simulink model "modello_completo_simulink2019b"  (R2019b)
settings: Solver=VariableStepAuto  StartTime=0.0  StopTime=30  RelTol=1e-3
undefined symbols (not defined in the file): a, a1, a2, AHRS_bias, AHRS_sample_time, AHRS_var, alpha1, alpha2, c, current, D, dead_zone_limit, DiscIntNeverNeededParam, DVL_sample_t, DVL_var1, DVL_var2, DVL_var3, gps_sample_t, H, IMU_sample_time, initial, INSP, Ki_bodypos1, Ki_bodypos2, Ki_bodypos3, Ki_bodypos4, Ki_bodypos5, Ki_depth1, Ki_depth2, Ki_depth3, Ki_depth4, Ki_depth5, Ki_latvel1, Ki_latvel2, Ki_latvel3, Ki_latvel4, Ki_latvel5, Ki_P1, Ki_P2, Ki_P3, Ki_P4, Ki_P5, Ki_R1, Ki_R2, Ki_R3, Ki_R4, Ki_R5, Ki_rel_or1, Ki_rel_or2, Ki_rel_or3, Ki_rel_or4, Ki_rel_or5, Ki_reldist1, Ki_reldist2, Ki_reldist3, Ki_reldist4, Ki_reldist5, Ki_surge1, Ki_surge2, Ki_surge3 ... (+66)
libraries: simulink x3
(part 4 of 5)

== system modello_completo_simulink2019b/Controller/POSIZIONAMENTO/PID_PITCH ==
  pitch_err : Inport
  EN6 : Inport  Port=2
  Constant : Constant  Value=0
  Discrete-Time Integrator : DiscreteIntegrator  ExternalReset=falling  SampleTime=0.1  ICPrevOutput=DiscIntNeverNeededParam  ICPrevScaledInput=DiscIntNeverNeededParam
  Display : Display
  Display1 : Display
  Gain : Gain  Gain=Kp_P1
  Gain2 : Gain  Gain=Ki_P1
  Sum : Sum  Inputs=++|
  Switch : Switch  Criteria=u2 > Threshold  Threshold=0.5
  tau_pitch : Outport
  wires:
  Switch/1 -> Gain/1, Gain2/1
  Constant/1 -> Switch/3
  EN6/1 -> Display/1, Switch/2, [EN6]
  pitch_err/1 -> Switch/1
  Gain/1 -> Sum/1
  Discrete-Time Integrator/1 -> Sum/2
  Sum/1 -> Display1/1, tau_pitch/1
  Gain2/1 -> Discrete-Time Integrator/1
  [EN6] -> Discrete-Time Integrator/2

== system modello_completo_simulink2019b/Controller/POSIZIONAMENTO/PID_ROLL  ==
  roll_err : Inport
  EN6 : Inport  Port=2
  Constant : Constant  Value=0
  Discrete-Time Integrator : DiscreteIntegrator  ExternalReset=falling  SampleTime=0.1  ICPrevOutput=DiscIntNeverNeededParam  ICPrevScaledInput=DiscIntNeverNeededParam
  Gain : Gain  Gain=Kp_R1
  Gain2 : Gain  Gain=Ki_R1
  Sum : Sum  Inputs=++|
  Switch : Switch  Criteria=u2 > Threshold  Threshold=0.5
  tau_roll : Outport
  wires:
  [EN6] -> Discrete-Time Integrator/2
  Switch/1 -> Gain/1, Gain2/1
  EN6/1 -> Switch/2, [EN6]
  roll_err/1 -> Switch/1
  Sum/1 -> tau_roll/1
  Gain2/1 -> Discrete-Time Integrator/1
  Gain/1 -> Sum/1
  Discrete-Time Integrator/1 -> Sum/2
  Constant/1 -> Switch/3

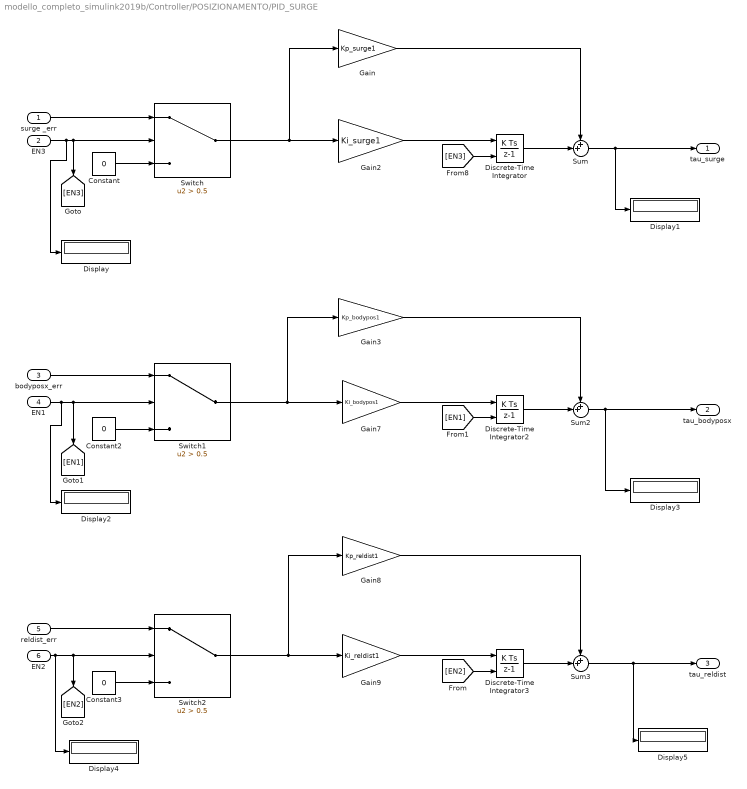
== system modello_completo_simulink2019b/Controller/POSIZIONAMENTO/PID_SURGE ==
  surge _err : Inport
  EN3 : Inport  Port=2
  bodyposx_err : Inport  Port=3
  EN1 : Inport  Port=4
  reldist_err : Inport  Port=5
  EN2 : Inport  Port=6
  Constant : Constant  Value=0
  Constant2 : Constant  Value=0
  Constant3 : Constant  Value=0
  Discrete-Time Integrator : DiscreteIntegrator  ExternalReset=falling  SampleTime=0.1  ICPrevOutput=DiscIntNeverNeededParam  ICPrevScaledInput=DiscIntNeverNeededParam
  Discrete-Time Integrator2 : DiscreteIntegrator  ExternalReset=falling  SampleTime=0.1  ICPrevOutput=DiscIntNeverNeededParam  ICPrevScaledInput=DiscIntNeverNeededParam
  Discrete-Time Integrator3 : DiscreteIntegrator  ExternalReset=falling  SampleTime=0.1  ICPrevOutput=DiscIntNeverNeededParam  ICPrevScaledInput=DiscIntNeverNeededParam
  Display{,1..5} (6 alike) : Display
  Gain : Gain  Gain=Kp_surge1
  Gain2 : Gain  Gain=Ki_surge1
  Gain3 : Gain  Gain=Kp_bodypos1
  Gain7 : Gain  Gain=Ki_bodypos1
  Gain8 : Gain  Gain=Kp_reldist1
  Gain9 : Gain  Gain=Ki_reldist1
  Sum : Sum  Inputs=++|
  Sum2 : Sum  Inputs=++|
  Sum3 : Sum  Inputs=++|
  Switch : Switch  Criteria=u2 > Threshold  Threshold=0.5
  Switch1 : Switch  Criteria=u2 > Threshold  Threshold=0.5
  Switch2 : Switch  Criteria=u2 > Threshold  Threshold=0.5
  tau_surge : Outport
  tau_bodyposx : Outport  Port=2
  tau_reldist : Outport  Port=3
  wires:
  Sum2/1 -> Display3/1, tau_bodyposx/1
  Gain9/1 -> Discrete-Time Integrator3/1
  EN2/1 -> Display4/1, [EN2], Switch2/2
  reldist_err/1 -> Switch2/1
  [EN2] -> Discrete-Time Integrator3/2
  Discrete-Time Integrator3/1 -> Sum3/2
  Switch2/1 -> Gain9/1, Gain8/1
  Sum3/1 -> Display5/1, tau_reldist/1
  Gain8/1 -> Sum3/1
  Constant3/1 -> Switch2/3
  [EN1] -> Discrete-Time Integrator2/2
  Switch1/1 -> Gain3/1, Gain7/1
  EN1/1 -> Display2/1, [EN1], Switch1/2
  bodyposx_err/1 -> Switch1/1
  Constant2/1 -> Switch1/3
  Gain3/1 -> Sum2/1
  Discrete-Time Integrator2/1 -> Sum2/2
  Gain7/1 -> Discrete-Time Integrator2/1
  Switch/1 -> Gain/1, Gain2/1
  EN3/1 -> Display/1, Switch/2, [EN3]
  surge _err/1 -> Switch/1
  Sum/1 -> Display1/1, tau_surge/1
  Gain2/1 -> Discrete-Time Integrator/1
  Discrete-Time Integrator/1 -> Sum/2
  [EN3] -> Discrete-Time Integrator/2
  Constant/1 -> Switch/3
  Gain/1 -> Sum/1

== system modello_completo_simulink2019b/Controller/POSIZIONAMENTO/PID_SWAY ==
  latvel_err : Inport
  EN4 : Inport  Port=2
  bodyposy_err : Inport  Port=3
  EN1 : Inport  Port=4
  Constant : Constant  Value=0
  Constant1 : Constant  Value=0
  Discrete-Time Integrator : DiscreteIntegrator  ExternalReset=falling  SampleTime=0.1  ICPrevOutput=DiscIntNeverNeededParam  ICPrevScaledInput=DiscIntNeverNeededParam
  Discrete-Time Integrator1 : DiscreteIntegrator  ExternalReset=falling  SampleTime=0.1  ICPrevOutput=DiscIntNeverNeededParam  ICPrevScaledInput=DiscIntNeverNeededParam
  Gain : Gain  Gain=Kp_latvel1
  Gain1 : Gain  Gain=Kp_bodypos1
  Gain2 : Gain  Gain=Ki_latvel1
  Gain4 : Gain  Gain=Ki_bodypos1
  Sum : Sum  Inputs=++|
  Sum1 : Sum  Inputs=++|
  Switch : Switch  Criteria=u2 > Threshold  Threshold=0.5
  Switch1 : Switch  Criteria=u2 > Threshold  Threshold=0.5
  tau_latvel : Outport
  tau_bodyposy : Outport  Port=2
  wires:
  Sum1/1 -> tau_bodyposy/1
  Switch1/1 -> Gain4/1, Gain1/1
  bodyposy_err/1 -> Switch1/1
  Constant1/1 -> Switch1/3
  EN1/1 -> [EN1], Switch1/2
  [EN1] -> Discrete-Time Integrator1/2
  Gain4/1 -> Discrete-Time Integrator1/1
  Gain1/1 -> Sum1/1
  Discrete-Time Integrator1/1 -> Sum1/2
  EN4/1 -> Switch/2, [EN4]
  [EN4] -> Discrete-Time Integrator/2
  latvel_err/1 -> Switch/1
  Gain2/1 -> Discrete-Time Integrator/1
  Discrete-Time Integrator/1 -> Sum/2
  Switch/1 -> Gain2/1, Gain/1
  Gain/1 -> Sum/1
  Sum/1 -> tau_latvel/1
  Constant/1 -> Switch/3

== system modello_completo_simulink2019b/Controller/POSIZIONAMENTO/PID_YAW ==
  yaw_err : Inport
  "EN8 " : Inport  Port=2
  rel_or_err : Inport  Port=3
  EN7 : Inport  Port=4
  Constant : Constant  Value=0
  Constant1 : Constant  Value=0
  Discrete-Time Integrator : DiscreteIntegrator  ExternalReset=falling  SampleTime=0.1  ICPrevOutput=DiscIntNeverNeededParam  ICPrevScaledInput=DiscIntNeverNeededParam
  Discrete-Time Integrator1 : DiscreteIntegrator  ExternalReset=falling  SampleTime=0.1  ICPrevOutput=DiscIntNeverNeededParam  ICPrevScaledInput=DiscIntNeverNeededParam
  Gain : Gain  Gain=Kp_yaw1
  Gain1 : Gain  Gain=Kp_rel_or1
  Gain2 : Gain  Gain=Ki_yaw1
  Gain3 : Gain  Gain=Ki_rel_or1
  Sum : Sum  Inputs=++|
  Sum1 : Sum  Inputs=++|
  Switch : Switch  Criteria=u2 > Threshold  Threshold=0.5
  Switch1 : Switch  Criteria=u2 > Threshold  Threshold=0.5
  tau_yaw : Outport
  tau_rel_or : Outport  Port=2
  wires:
  Gain1/1 -> Sum1/1
  Gain3/1 -> Discrete-Time Integrator1/1
  Constant1/1 -> Switch1/3
  Sum1/1 -> tau_rel_or/1
  Switch1/1 -> Gain3/1, Gain1/1
  EN7/1 -> Switch1/2, [EN7]
  rel_or_err/1 -> Switch1/1
  [EN7] -> Discrete-Time Integrator1/2
  Discrete-Time Integrator1/1 -> Sum1/2
  [EN8] -> Discrete-Time Integrator/2
  Gain2/1 -> Discrete-Time Integrator/1
  Constant/1 -> Switch/3
  "EN8 "/1 -> Switch/2, [EN8]
  Gain/1 -> Sum/1
  yaw_err/1 -> Switch/1
  Switch/1 -> Gain2/1, Gain/1
  Discrete-Time Integrator/1 -> Sum/2
  Sum/1 -> tau_yaw/1

== system modello_completo_simulink2019b/Controller/ROTAZIONE IN PROFONDITA'/PID_HEAVE ==
  depth_err : Inport
  EN5 : Inport  Port=2
  Constant : Constant  Value=0
  Discrete-Time Integrator : DiscreteIntegrator  ExternalReset=falling  SampleTime=0.1  ICPrevOutput=DiscIntNeverNeededParam  ICPrevScaledInput=DiscIntNeverNeededParam
  Gain : Gain  Gain=Kp_depth5
  Gain2 : Gain  Gain=Ki_depth5
  Sum : Sum  Inputs=++|
  Switch : Switch  Criteria=u2 > Threshold  Threshold=0.5
  tau_depth : Outport
  wires:
  Gain/1 -> Sum/1
  Discrete-Time Integrator/1 -> Sum/2
  Constant/1 -> Switch/3
  Switch/1 -> Gain/1, Gain2/1
  depth_err/1 -> Switch/1
  Sum/1 -> tau_depth/1
  Gain2/1 -> Discrete-Time Integrator/1
  EN5/1 -> [EN5], Switch/2
  [EN5] -> Discrete-Time Integrator/2

== system modello_completo_simulink2019b/Controller/ROTAZIONE IN PROFONDITA'/PID_PITCH ==
  pitch_err : Inport
  EN6 : Inport  Port=2
  Constant : Constant  Value=0
  Discrete-Time Integrator : DiscreteIntegrator  ExternalReset=falling  SampleTime=0.1  ICPrevOutput=DiscIntNeverNeededParam  ICPrevScaledInput=DiscIntNeverNeededParam
  Gain : Gain  Gain=Kp_P5
  Gain2 : Gain  Gain=Ki_P5
  Sum : Sum  Inputs=++|
  Switch : Switch  Criteria=u2 > Threshold  Threshold=0.5
  tau_pitch : Outport
  wires:
  [EN6] -> Discrete-Time Integrator/2
  Gain2/1 -> Discrete-Time Integrator/1
  Sum/1 -> tau_pitch/1
  Discrete-Time Integrator/1 -> Sum/2
  Gain/1 -> Sum/1
  pitch_err/1 -> Switch/1
  EN6/1 -> [EN6], Switch/2
  Constant/1 -> Switch/3
  Switch/1 -> Gain2/1, Gain/1

== system modello_completo_simulink2019b/Controller/ROTAZIONE IN PROFONDITA'/PID_ROLL  ==
  roll_err : Inport
  EN6 : Inport  Port=2
  Constant : Constant  Value=0
  Discrete-Time Integrator : DiscreteIntegrator  ExternalReset=falling  SampleTime=0.1  ICPrevOutput=DiscIntNeverNeededParam  ICPrevScaledInput=DiscIntNeverNeededParam
  Gain : Gain  Gain=Kp_R5
  Gain2 : Gain  Gain=Ki_R5
  Sum : Sum  Inputs=++|
  Switch : Switch  Criteria=u2 > Threshold  Threshold=0.5
  tau_roll : Outport
  wires:
  Constant/1 -> Switch/3
  Discrete-Time Integrator/1 -> Sum/2
  Gain/1 -> Sum/1
  Gain2/1 -> Discrete-Time Integrator/1
  Sum/1 -> tau_roll/1
  roll_err/1 -> Switch/1
  EN6/1 -> [EN6], Switch/2
  Switch/1 -> Gain2/1, Gain/1
  [EN6] -> Discrete-Time Integrator/2

== system modello_completo_simulink2019b/Controller/ROTAZIONE IN PROFONDITA'/PID_SURGE ==
  surge _err : Inport
  EN3 : Inport  Port=2
  bodyposx_err : Inport  Port=3
  EN1 : Inport  Port=4
  reldist_err : Inport  Port=5
  EN2 : Inport  Port=6
  Constant : Constant  Value=0
  Constant2 : Constant  Value=0
  Constant3 : Constant  Value=0
  Discrete-Time Integrator : DiscreteIntegrator  ExternalReset=falling  SampleTime=0.1  ICPrevOutput=DiscIntNeverNeededParam  ICPrevScaledInput=DiscIntNeverNeededParam
  Discrete-Time Integrator2 : DiscreteIntegrator  ExternalReset=falling  SampleTime=0.1  ICPrevOutput=DiscIntNeverNeededParam  ICPrevScaledInput=DiscIntNeverNeededParam
  Discrete-Time Integrator3 : DiscreteIntegrator  ExternalReset=falling  SampleTime=0.1  ICPrevOutput=DiscIntNeverNeededParam  ICPrevScaledInput=DiscIntNeverNeededParam
  Gain : Gain  Gain=Kp_surge5
  Gain2 : Gain  Gain=Ki_surge5
  Gain3 : Gain  Gain=Kp_bodypos5
  Gain7 : Gain  Gain=Ki_bodypos5
  Gain8 : Gain  Gain=Kp_reldist5
  Gain9 : Gain  Gain=Ki_reldist5
  Sum : Sum  Inputs=++|
  Sum2 : Sum  Inputs=++|
  Sum3 : Sum  Inputs=++|
  Switch : Switch  Criteria=u2 > Threshold  Threshold=0.5
  Switch1 : Switch  Criteria=u2 > Threshold  Threshold=0.5
  Switch2 : Switch  Criteria=u2 > Threshold  Threshold=0.5
  tau_surge : Outport
  tau_bodyposx : Outport  Port=2
  tau_reldist : Outport  Port=3
  wires:
  Gain/1 -> Sum/1
  Constant/1 -> Switch/3
  [EN3] -> Discrete-Time Integrator/2
  Discrete-Time Integrator/1 -> Sum/2
  Gain2/1 -> Discrete-Time Integrator/1
  Sum/1 -> tau_surge/1
  surge _err/1 -> Switch/1
  EN3/1 -> [EN3], Switch/2
  Switch/1 -> Gain2/1, Gain/1
  Gain7/1 -> Discrete-Time Integrator2/1
  Discrete-Time Integrator2/1 -> Sum2/2
  Gain3/1 -> Sum2/1
  Constant2/1 -> Switch1/3
  bodyposx_err/1 -> Switch1/1
  EN1/1 -> Switch1/2, [EN1]
  Switch1/1 -> Gain7/1, Gain3/1
  [EN1] -> Discrete-Time Integrator2/2
  Constant3/1 -> Switch2/3
  Gain8/1 -> Sum3/1
  Sum3/1 -> tau_reldist/1
  Switch2/1 -> Gain8/1, Gain9/1
  Discrete-Time Integrator3/1 -> Sum3/2
  [EN2] -> Discrete-Time Integrator3/2
  reldist_err/1 -> Switch2/1
  EN2/1 -> Switch2/2, [EN2]
  Gain9/1 -> Discrete-Time Integrator3/1
  Sum2/1 -> tau_bodyposx/1

== system modello_completo_simulink2019b/Controller/ROTAZIONE IN PROFONDITA'/PID_SWAY ==
  latvel_err : Inport
  EN4 : Inport  Port=2
  bodyposy_err : Inport  Port=3
  EN1 : Inport  Port=4
  Constant : Constant  Value=0
  Constant1 : Constant  Value=0
  Discrete-Time Integrator : DiscreteIntegrator  ExternalReset=falling  SampleTime=0.1  ICPrevOutput=DiscIntNeverNeededParam  ICPrevScaledInput=DiscIntNeverNeededParam
  Discrete-Time Integrator1 : DiscreteIntegrator  ExternalReset=falling  SampleTime=0.1  ICPrevOutput=DiscIntNeverNeededParam  ICPrevScaledInput=DiscIntNeverNeededParam
  Gain : Gain  Gain=Kp_latvel5
  Gain1 : Gain  Gain=Kp_bodypos5
  Gain2 : Gain  Gain=Ki_latvel5
  Gain4 : Gain  Gain=Ki_bodypos5
  Sum : Sum  Inputs=++|
  Sum1 : Sum  Inputs=++|
  Switch : Switch  Criteria=u2 > Threshold  Threshold=0.5
  Switch1 : Switch  Criteria=u2 > Threshold  Threshold=0.5
  tau_latvel : Outport
  tau_bodyposy : Outport  Port=2
  wires:
  Constant/1 -> Switch/3
  Sum/1 -> tau_latvel/1
  Gain/1 -> Sum/1
  Switch/1 -> Gain/1, Gain2/1
  Discrete-Time Integrator/1 -> Sum/2
  Gain2/1 -> Discrete-Time Integrator/1
  latvel_err/1 -> Switch/1
  [EN4] -> Discrete-Time Integrator/2
  EN4/1 -> [EN4], Switch/2
  Discrete-Time Integrator1/1 -> Sum1/2
  Gain1/1 -> Sum1/1
  Gain4/1 -> Discrete-Time Integrator1/1
  [EN1] -> Discrete-Time Integrator1/2
  EN1/1 -> Switch1/2, [EN1]
  Constant1/1 -> Switch1/3
  bodyposy_err/1 -> Switch1/1
  Switch1/1 -> Gain1/1, Gain4/1
  Sum1/1 -> tau_bodyposy/1

== system modello_completo_simulink2019b/Controller/ROTAZIONE IN PROFONDITA'/PID_YAW ==
  yaw_err : Inport
  "EN8 " : Inport  Port=2
  rel_or_err : Inport  Port=3
  EN7 : Inport  Port=4
  Constant : Constant  Value=0
  Constant1 : Constant  Value=0
  Discrete-Time Integrator : DiscreteIntegrator  ExternalReset=falling  SampleTime=0.1  ICPrevOutput=DiscIntNeverNeededParam  ICPrevScaledInput=DiscIntNeverNeededParam
  Discrete-Time Integrator1 : DiscreteIntegrator  ExternalReset=falling  SampleTime=0.1  ICPrevOutput=DiscIntNeverNeededParam  ICPrevScaledInput=DiscIntNeverNeededParam
  Gain : Gain  Gain=Kp_yaw5
  Gain1 : Gain  Gain=Kp_rel_or5
  Gain2 : Gain  Gain=Ki_yaw5
  Gain3 : Gain  Gain=Ki_rel_or5
  Sum : Sum  Inputs=++|
  Sum1 : Sum  Inputs=++|
  Switch : Switch  Criteria=u2 > Threshold  Threshold=0.5
  Switch1 : Switch  Criteria=u2 > Threshold  Threshold=0.5
  tau_yaw : Outport
  tau_rel_or : Outport  Port=2
  wires:
  Sum/1 -> tau_yaw/1
  Discrete-Time Integrator/1 -> Sum/2
  Switch/1 -> Gain/1, Gain2/1
  yaw_err/1 -> Switch/1
  Gain/1 -> Sum/1
  "EN8 "/1 -> [EN8], Switch/2
  Constant/1 -> Switch/3
  Gain2/1 -> Discrete-Time Integrator/1
  [EN8] -> Discrete-Time Integrator/2
  Discrete-Time Integrator1/1 -> Sum1/2
  [EN7] -> Discrete-Time Integrator1/2
  rel_or_err/1 -> Switch1/1
  EN7/1 -> [EN7], Switch1/2
  Switch1/1 -> Gain1/1, Gain3/1
  Sum1/1 -> tau_rel_or/1
  Constant1/1 -> Switch1/3
  Gain3/1 -> Discrete-Time Integrator1/1
  Gain1/1 -> Sum1/1

== system modello_completo_simulink2019b/Controller/ROTAZIONE IN SUPERFICIE/PID_HEAVE ==
  depth_err : Inport
  EN5 : Inport  Port=2
  Constant : Constant  Value=0
  Discrete-Time Integrator : DiscreteIntegrator  ExternalReset=falling  SampleTime=0.1  ICPrevOutput=DiscIntNeverNeededParam  ICPrevScaledInput=DiscIntNeverNeededParam
  Gain : Gain  Gain=Kp_depth3
  Gain2 : Gain  Gain=Ki_depth3
  Sum : Sum  Inputs=++|
  Switch : Switch  Criteria=u2 > Threshold  Threshold=0.5
  tau_depth : Outport
  wires:
  Gain/1 -> Sum/1
  Discrete-Time Integrator/1 -> Sum/2
  Constant/1 -> Switch/3
  Switch/1 -> Gain/1, Gain2/1
  depth_err/1 -> Switch/1
  Sum/1 -> tau_depth/1
  Gain2/1 -> Discrete-Time Integrator/1
  EN5/1 -> [EN5], Switch/2
  [EN5] -> Discrete-Time Integrator/2

== system modello_completo_simulink2019b/Controller/ROTAZIONE IN SUPERFICIE/PID_PITCH ==
  pitch_err : Inport
  EN6 : Inport  Port=2
  Constant : Constant  Value=0
  Discrete-Time Integrator : DiscreteIntegrator  ExternalReset=falling  SampleTime=0.1  ICPrevOutput=DiscIntNeverNeededParam  ICPrevScaledInput=DiscIntNeverNeededParam
  Gain : Gain  Gain=Kp_P3
  Gain2 : Gain  Gain=Ki_P3
  Sum : Sum  Inputs=++|
  Switch : Switch  Criteria=u2 > Threshold  Threshold=0.5
  tau_pitch : Outport
  wires:
  [EN6] -> Discrete-Time Integrator/2
  Gain2/1 -> Discrete-Time Integrator/1
  Sum/1 -> tau_pitch/1
  Discrete-Time Integrator/1 -> Sum/2
  Gain/1 -> Sum/1
  pitch_err/1 -> Switch/1
  EN6/1 -> [EN6], Switch/2
  Constant/1 -> Switch/3
  Switch/1 -> Gain2/1, Gain/1

== system modello_completo_simulink2019b/Controller/ROTAZIONE IN SUPERFICIE/PID_ROLL  ==
  roll_err : Inport
  EN6 : Inport  Port=2
  Constant : Constant  Value=0
  Discrete-Time Integrator : DiscreteIntegrator  ExternalReset=falling  SampleTime=0.1  ICPrevOutput=DiscIntNeverNeededParam  ICPrevScaledInput=DiscIntNeverNeededParam
  Gain : Gain  Gain=Kp_R3
  Gain2 : Gain  Gain=Ki_R3
  Sum : Sum  Inputs=++|
  Switch : Switch  Criteria=u2 > Threshold  Threshold=0.5
  tau_roll : Outport
  wires:
  Constant/1 -> Switch/3
  Discrete-Time Integrator/1 -> Sum/2
  Gain/1 -> Sum/1
  Gain2/1 -> Discrete-Time Integrator/1
  Sum/1 -> tau_roll/1
  roll_err/1 -> Switch/1
  EN6/1 -> [EN6], Switch/2
  Switch/1 -> Gain2/1, Gain/1
  [EN6] -> Discrete-Time Integrator/2

== system modello_completo_simulink2019b/Controller/ROTAZIONE IN SUPERFICIE/PID_SURGE ==
  surge _err : Inport
  EN3 : Inport  Port=2
  bodyposx_err : Inport  Port=3
  EN1 : Inport  Port=4
  reldist_err : Inport  Port=5
  EN2 : Inport  Port=6
  Constant : Constant  Value=0
  Constant2 : Constant  Value=0
  Constant3 : Constant  Value=0
  Discrete-Time Integrator : DiscreteIntegrator  ExternalReset=falling  SampleTime=0.1  ICPrevOutput=DiscIntNeverNeededParam  ICPrevScaledInput=DiscIntNeverNeededParam
  Discrete-Time Integrator2 : DiscreteIntegrator  ExternalReset=falling  SampleTime=0.1  ICPrevOutput=DiscIntNeverNeededParam  ICPrevScaledInput=DiscIntNeverNeededParam
  Discrete-Time Integrator3 : DiscreteIntegrator  ExternalReset=falling  SampleTime=0.1  ICPrevOutput=DiscIntNeverNeededParam  ICPrevScaledInput=DiscIntNeverNeededParam
  Gain : Gain  Gain=Kp_surge3
  Gain2 : Gain  Gain=Ki_surge3
  Gain3 : Gain  Gain=Kp_bodypos3
  Gain7 : Gain  Gain=Ki_bodypos3
  Gain8 : Gain  Gain=Kp_reldist3
  Gain9 : Gain  Gain=Ki_reldist3
  Sum : Sum  Inputs=++|
  Sum2 : Sum  Inputs=++|
  Sum3 : Sum  Inputs=++|
  Switch : Switch  Criteria=u2 > Threshold  Threshold=0.5
  Switch1 : Switch  Criteria=u2 > Threshold  Threshold=0.5
  Switch2 : Switch  Criteria=u2 > Threshold  Threshold=0.5
  tau_surge : Outport
  tau_bodyposx : Outport  Port=2
  tau_reldist : Outport  Port=3
  wires:
  Gain/1 -> Sum/1
  Constant/1 -> Switch/3
  [EN3] -> Discrete-Time Integrator/2
  Discrete-Time Integrator/1 -> Sum/2
  Gain2/1 -> Discrete-Time Integrator/1
  Sum/1 -> tau_surge/1
  surge _err/1 -> Switch/1
  EN3/1 -> [EN3], Switch/2
  Switch/1 -> Gain2/1, Gain/1
  Gain7/1 -> Discrete-Time Integrator2/1
  Discrete-Time Integrator2/1 -> Sum2/2
  Gain3/1 -> Sum2/1
  Constant2/1 -> Switch1/3
  bodyposx_err/1 -> Switch1/1
  EN1/1 -> Switch1/2, [EN1]
  Switch1/1 -> Gain7/1, Gain3/1
  [EN1] -> Discrete-Time Integrator2/2
  Constant3/1 -> Switch2/3
  Gain8/1 -> Sum3/1
  Sum3/1 -> tau_reldist/1
  Switch2/1 -> Gain8/1, Gain9/1
  Discrete-Time Integrator3/1 -> Sum3/2
  [EN2] -> Discrete-Time Integrator3/2
  reldist_err/1 -> Switch2/1
  EN2/1 -> Switch2/2, [EN2]
  Gain9/1 -> Discrete-Time Integrator3/1
  Sum2/1 -> tau_bodyposx/1

== system modello_completo_simulink2019b/Controller/ROTAZIONE IN SUPERFICIE/PID_SWAY ==
  latvel_err : Inport
  EN4 : Inport  Port=2
  bodyposy_err : Inport  Port=3
  EN1 : Inport  Port=4
  Constant : Constant  Value=0
  Constant1 : Constant  Value=0
  Discrete-Time Integrator : DiscreteIntegrator  ExternalReset=falling  SampleTime=0.1  ICPrevOutput=DiscIntNeverNeededParam  ICPrevScaledInput=DiscIntNeverNeededParam
  Discrete-Time Integrator1 : DiscreteIntegrator  ExternalReset=falling  SampleTime=0.1  ICPrevOutput=DiscIntNeverNeededParam  ICPrevScaledInput=DiscIntNeverNeededParam
  Gain : Gain  Gain=Kp_latvel3
  Gain1 : Gain  Gain=Kp_bodypos3
  Gain2 : Gain  Gain=Ki_latvel3
  Gain4 : Gain  Gain=Ki_bodypos3
  Sum : Sum  Inputs=++|
  Sum1 : Sum  Inputs=++|
  Switch : Switch  Criteria=u2 > Threshold  Threshold=0.5
  Switch1 : Switch  Criteria=u2 > Threshold  Threshold=0.5
  tau_latvel : Outport
  tau_bodyposy : Outport  Port=2
  wires:
  Constant/1 -> Switch/3
  Sum/1 -> tau_latvel/1
  Gain/1 -> Sum/1
  Switch/1 -> Gain/1, Gain2/1
  Discrete-Time Integrator/1 -> Sum/2
  Gain2/1 -> Discrete-Time Integrator/1
  latvel_err/1 -> Switch/1
  [EN4] -> Discrete-Time Integrator/2
  EN4/1 -> [EN4], Switch/2
  Discrete-Time Integrator1/1 -> Sum1/2
  Gain1/1 -> Sum1/1
  Gain4/1 -> Discrete-Time Integrator1/1
  [EN1] -> Discrete-Time Integrator1/2
  EN1/1 -> Switch1/2, [EN1]
  Constant1/1 -> Switch1/3
  bodyposy_err/1 -> Switch1/1
  Switch1/1 -> Gain1/1, Gain4/1
  Sum1/1 -> tau_bodyposy/1

== system modello_completo_simulink2019b/Controller/ROTAZIONE IN SUPERFICIE/PID_YAW ==
  yaw_err : Inport
  "EN8 " : Inport  Port=2
  rel_or_err : Inport  Port=3
  EN7 : Inport  Port=4
  Constant : Constant  Value=0
  Constant1 : Constant  Value=0
  Discrete-Time Integrator : DiscreteIntegrator  ExternalReset=falling  SampleTime=0.1  ICPrevOutput=DiscIntNeverNeededParam  ICPrevScaledInput=DiscIntNeverNeededParam
  Discrete-Time Integrator1 : DiscreteIntegrator  ExternalReset=falling  SampleTime=0.1  ICPrevOutput=DiscIntNeverNeededParam  ICPrevScaledInput=DiscIntNeverNeededParam
  Gain : Gain  Gain=Kp_yaw3
  Gain1 : Gain  Gain=Kp_rel_or3
  Gain2 : Gain  Gain=Ki_yaw3
  Gain3 : Gain  Gain=Ki_rel_or3
  Sum : Sum  Inputs=++|
  Sum1 : Sum  Inputs=++|
  Switch : Switch  Criteria=u2 > Threshold  Threshold=0.5
  Switch1 : Switch  Criteria=u2 > Threshold  Threshold=0.5
  tau_yaw : Outport
  tau_rel_or : Outport  Port=2
  wires:
  Sum/1 -> tau_yaw/1
  Discrete-Time Integrator/1 -> Sum/2
  Switch/1 -> Gain/1, Gain2/1
  yaw_err/1 -> Switch/1
  Gain/1 -> Sum/1
  "EN8 "/1 -> [EN8], Switch/2
  Constant/1 -> Switch/3
  Gain2/1 -> Discrete-Time Integrator/1
  [EN8] -> Discrete-Time Integrator/2
  Discrete-Time Integrator1/1 -> Sum1/2
  [EN7] -> Discrete-Time Integrator1/2
  rel_or_err/1 -> Switch1/1
  EN7/1 -> [EN7], Switch1/2
  Switch1/1 -> Gain1/1, Gain3/1
  Sum1/1 -> tau_rel_or/1
  Constant1/1 -> Switch1/3
  Gain3/1 -> Discrete-Time Integrator1/1
  Gain1/1 -> Sum1/1

== system modello_completo_simulink2019b/Env. & Sensor Model/AHRS SENSOR/Accelerometer ==
  note: Noise Density: < 0.14 mg/√Hz
  In1 : Inport
  Band-Limited White Noise : simulink/Sources/Band-Limited White Noise  Cov=acc_noise  Ts=IMU_sample_time  seed=acc_seed
  Bias : Bias  Bias=0.0
  Noise : Gain
  Sum : Sum  Inputs=|++
  lin_acc : Outport
  wires:
  Band-Limited White Noise/1 -> Noise/1
  Sum/1 -> lin_acc/1
  Bias/1 -> Sum/1
  In1/1 -> Bias/1
  Noise/1 -> Sum/2

== system modello_completo_simulink2019b/Env. & Sensor Model/AHRS SENSOR/Gyroscope ==
  note: Noise Density: 0.0035 °/s √Hz
  In1 : Inport
  Band-Limited White Noise : simulink/Sources/Band-Limited White Noise  Cov=gyro_noise  Ts=IMU_sample_time  seed=gyro_seed
  Bias : Bias  Bias=0.0
  Noise : Gain
  Sum : Sum  Inputs=|++
  ang_vel : Outport
  wires:
  Band-Limited White Noise/1 -> Noise/1
  Sum/1 -> ang_vel/1
  Bias/1 -> Sum/1
  In1/1 -> Bias/1
  Noise/1 -> Sum/2

== system modello_completo_simulink2019b/Env. & Sensor Model/AHRS SENSOR/Magnetometer ==
  note: Noise Density: 140 μGauss/√Hz
  In1 : Inport
  Band-Limited White Noise : simulink/Sources/Band-Limited White Noise  Cov=magn_noise  Ts=IMU_sample_time  seed=[31]
  Bias : Bias  Bias=0.0
  Sum : Sum  Inputs=|++
  m : Outport
  wires:
  Band-Limited White Noise/1 -> Sum/2
  Sum/1 -> m/1
  Bias/1 -> Sum/1
  In1/1 -> Bias/1

== system modello_completo_simulink2019b/Env. & Sensor Model/DVL SENSOR/Subsystem ==
  In1 : Inport
  Abs : Abs
  Noise : Gain
  Random Number : RandomNumber  Variance=DVL_var3  Seed=1  SampleTime=DVL_sample_t
  Random Number1 : RandomNumber  Variance=DVL_var2  Seed=2  SampleTime=DVL_sample_t
  Random Number2 : RandomNumber  Variance=DVL_var1  Seed=3  SampleTime=DVL_sample_t
  Switch2 : Switch  Criteria=u2 > Threshold  Threshold=2
  Switch3 : Switch  Criteria=u2 > Threshold  Threshold=4
  Out1 : Outport
  wires:
  Switch3/1 -> Switch2/1
  Random Number1/1 -> Switch3/3
  Random Number2/1 -> Switch2/3
  In1/1 -> Noise/1
  Switch2/1 -> Out1/1
  Random Number/1 -> Switch3/1
  Abs/1 -> Switch3/2, Switch2/2
  Noise/1 -> Abs/1

== system modello_completo_simulink2019b/Env. & Sensor Model/DVL SENSOR/Subsystem1 ==
  In1 : Inport
  Abs : Abs
  Noise : Gain
  Random Number : RandomNumber  Variance=DVL_var3  Seed=4  SampleTime=DVL_sample_t
  Random Number1 : RandomNumber  Variance=DVL_var2  Seed=5  SampleTime=DVL_sample_t
  Random Number2 : RandomNumber  Variance=DVL_var1  Seed=2  SampleTime=DVL_sample_t
  Switch2 : Switch  Criteria=u2 > Threshold  Threshold=2
  Switch3 : Switch  Criteria=u2 > Threshold  Threshold=4
  Out1 : Outport
  wires:
  Switch3/1 -> Switch2/1
  Random Number1/1 -> Switch3/3
  Random Number2/1 -> Switch2/3
  In1/1 -> Noise/1
  Switch2/1 -> Out1/1
  Random Number/1 -> Switch3/1
  Abs/1 -> Switch3/2, Switch2/2
  Noise/1 -> Abs/1

== system modello_completo_simulink2019b/Env. & Sensor Model/DVL SENSOR/Subsystem2 ==
  In1 : Inport
  Abs : Abs
  Gain : Gain
  Random Number : RandomNumber  Variance=DVL_var3  Seed=7  SampleTime=DVL_sample_t
  Random Number1 : RandomNumber  Variance=DVL_var2  Seed=2  SampleTime=DVL_sample_t
  Random Number2 : RandomNumber  Variance=DVL_var1  Seed=1  SampleTime=DVL_sample_t
  Switch2 : Switch  Criteria=u2 > Threshold  Threshold=2
  Switch3 : Switch  Criteria=u2 > Threshold  Threshold=4
  Out1 : Outport
  wires:
  Switch3/1 -> Switch2/1
  Random Number1/1 -> Switch3/3
  Random Number2/1 -> Switch2/3
  In1/1 -> Gain/1
  Switch2/1 -> Out1/1
  Random Number/1 -> Switch3/1
  Abs/1 -> Switch3/2, Switch2/2
  Gain/1 -> Abs/1

== system modello_completo_simulink2019b/Env. & Sensor Model/GPS SENSOR/Add noiose ==
  In1 : Inport
  In2 : Inport  Port=2
  Bus Creator : BusCreator  Inputs=2
  Noise GPS : Constant
  Product : Product
  Product1 : Product
  Random Number : RandomNumber  Variance=2  SampleTime=1
  Random Number1 : RandomNumber  Variance=2  Seed=332  SampleTime=1
  Sum2 : Sum  Inputs=|++
  Sum3 : Sum  Inputs=|++
  Out1 : Outport
  wires:
  In2/1 -> Sum3/2  "y in"
  Bus Creator/1 -> Out1/1  "out"
  In1/1 -> Sum2/1  "x in"
  Random Number/1 -> Product/1  "noise x"
  Random Number1/1 -> Product1/2  "noise y"
  Sum2/1 -> Bus Creator/1  "x"
  Sum3/1 -> Bus Creator/2  "y"
  Product/1 -> Sum2/2
  Product1/1 -> Sum3/1
  Noise GPS/1 -> Product1/1, Product/2

== system modello_completo_simulink2019b/Env. & Sensor Model/GPS SENSOR/Control state ==
  In1 : Inport
  AND : Logic  IconShape=distinctive  AllPortsSameDT=off  OutDataTypeStr=boolean
  Data Type Conversion : DataTypeConversion  OutDataTypeStr=double
  ENABLE GPS : Constant
  Zero-Order Hold : ZeroOrderHold  SampleTime=gps_sample_t
  Flag enable gps : Outport
  wires:
  ENABLE GPS/1 -> AND/2
  In1/1 -> AND/1
  AND/1 -> Data Type Conversion/1
  Data Type Conversion/1 -> Zero-Order Hold/1
  Zero-Order Hold/1 -> Flag enable gps/1

== system modello_completo_simulink2019b/Env. & Sensor Model/Sonar sensor/Control ==
  In1 : Inport
  Demux2 : Demux  Outputs=5
  Terminator{,1..4} (5 alike) : Terminator
  wires:
  Demux2/1 -> Terminator/1  "1"
  Demux2/5 -> Terminator4/1  "5"
  Demux2/2 -> Terminator1/1  "2"
  Demux2/4 -> Terminator3/1  "4"
  In1/1 -> Demux2/1
  Demux2/3 -> Terminator2/1  "3"

== system modello_completo_simulink2019b/Env. & Sensor Model/Sonar sensor/Noises ==
  Mux : Mux  Inputs=s_data.num
  Noise : Gain
  Random Number : RandomNumber  Mean=s_data.bias  Variance=s_data.noise^2  Seed=1  SampleTime=s_data.smpl  VectorParams1D=off
  Random Number1 : RandomNumber  Mean=s_data.bias  Variance=s_data.noise^2  Seed=2  SampleTime=s_data.smpl  VectorParams1D=off
  Random Number2 : RandomNumber  Mean=s_data.bias  Variance=s_data.noise^2  Seed=3  SampleTime=s_data.smpl  VectorParams1D=off
  Random Number3 : RandomNumber  Mean=s_data.bias  Variance=s_data.noise^2  Seed=4  SampleTime=s_data.smpl  VectorParams1D=off
  Random Number4 : RandomNumber  Mean=s_data.bias  Variance=s_data.noise^2  Seed=5  SampleTime=s_data.smpl  VectorParams1D=off
  Noises : Outport  SampleTime=s_data.smpl
  wires:
  Mux/1 -> Noise/1
  Random Number/1 -> Mux/1
  Random Number1/1 -> Mux/2
  Random Number2/1 -> Mux/3
  Random Number3/1 -> Mux/4
  Random Number4/1 -> Mux/5
  Noise/1 -> Noises/1

== system modello_completo_simulink2019b/Navigation1/Relative estimation/Sonar trigger ==
  In1 : Inport
  Demux : Demux  Outputs=[5 5]
  MATLAB Function : MATLAB Function  TreatAsAtomicUnit=on
  Scope2 : Scope
  Sum : Sum  Inputs=|+-
  Terminator : Terminator
  prev_sonar : Memory  InitialCondition=zeros(5,1)
  Out2 : Outport
  wires:
  Sum/1 -> MATLAB Function/2(sum)
  prev_sonar/1 -> Sum/2
  MATLAB Function/1(pulse) -> Out2/1, Scope2/1
  Demux/2 -> Terminator/1
  MATLAB Function/2(prev) -> prev_sonar/1
  In1/1 -> Demux/1
  Demux/1 -> MATLAB Function/1(sonar), Sum/1

== system modello_completo_simulink2019b/Navigation1/Relative estimation/Subsystem ==
  Sonar : Inport
  Orientation : Inport  Port=2
  Trigger : TriggerPort  VariantControl=Variant  PortDimensions=1
  Demux : Demux  Outputs=[5 5]
  Display : Display
  Display1 : Display
  MATLAB Function9 : MATLAB Function  TreatAsAtomicUnit=on
  Terminator : Terminator
  Rel_distance : Outport  PortDimensions=1
  Rel_angle : Outport  Port=2  PortDimensions=1
  flag_sonar : Outport  Port=3  PortDimensions=1
  wires:
  Sonar/1 -> Demux/1, MATLAB Function9/1(sonar)
  MATLAB Function9/3(flag_sonar) -> Display/1, flag_sonar/1
  Orientation/1 -> MATLAB Function9/2(orientation)
  MATLAB Function9/2(alpha) -> Rel_angle/1
  MATLAB Function9/1(distance) -> Rel_distance/1
  Demux/1 -> Terminator/1
  Demux/2 -> Display1/1

== system modello_completo_simulink2019b/Navigation1/z_EKF/EXTENDED KALMAN FILTER ==
  dT : Inport
  init : Inport  Port=2
  P0 : Inport  Port=3
  meas_pos : Inport  Port=4
  GPS_flag : Inport  Port=5
  meas_depth : Inport  Port=6
  orientation : Inport  Port=7
  dvl : Inport  Port=8
  ahrs_flag : Inport  Port=9
  Trigger : TriggerPort  VariantControl=Variant  PortDimensions=1
  "Correzione " : MATLAB Function  TreatAsAtomicUnit=on
  Demux : Demux  Outputs=[2 1]
  P : Memory  InitialCondition=zeros(3)  InheritSampleTime=on  StateName=P_pos
  Predizione : MATLAB Function  TreatAsAtomicUnit=on
  Scope : Scope
  hat_ : Memory  InitialCondition=zeros(3,1)  InheritSampleTime=on  StateName=P_pos
  previous_pos : Memory  InitialCondition=zeros(2,1)  InheritSampleTime=on  StateName=P_pos
  hat_pos : Outport
  hat_depth : Outport  Port=2
  wires:
  P/1 -> Predizione/1("P ")
  "Correzione "/2(P) -> P/1, Scope/1
  "Correzione "/1(prev_pos) -> previous_pos/1
  hat_/1 -> Predizione/2("hat ")
  "Correzione "/3(hat) -> Demux/1, hat_/1
  previous_pos/1 -> "Correzione "/1("prev_pos ")
  init/1 -> Predizione/7(init)
  orientation/1 -> Predizione/4(orientation)
  dT/1 -> Predizione/3(dT)
  dvl/1 -> Predizione/5(dvl)
  ahrs_flag/1 -> Predizione/6(ahrs_flag)
  P0/1 -> Predizione/8(P0)
  Predizione/1(P) -> "Correzione "/2("P ")
  Predizione/2(hat) -> "Correzione "/3("hat ")
  meas_pos/1 -> "Correzione "/4(meas_pos)
  GPS_flag/1 -> "Correzione "/5(GPS_flag)
  Demux/1 -> hat_pos/1
  Demux/2 -> hat_depth/1
  meas_depth/1 -> "Correzione "/6(meas_depth)

== system modello_completo_simulink2019b/Navigation1/z_EKF/Trigger & Init ==
  meas_depth : Inport
  "meas_pos " : Inport  Port=2
  AND : Logic  IconShape=distinctive  AllPortsSameDT=off  OutDataTypeStr=boolean
  Depth trigger : Subsystem
  Initialization : Subsystem
  Scope{,1..3} (4 alike) : Scope
  pulse : Outport
  dT : Outport  Port=2
  init : Outport  Port=3
  P0 : Outport  Port=4
  wires:
  meas_depth/1 -> Depth trigger/1(Meas_depth), Initialization/1(Meas_depth)
  Depth trigger/2(Pulse) -> AND/1, Scope2/1
  "meas_pos "/1 -> Initialization/2(Meas_pos)
  Initialization/2(init) -> init/1, Scope3/1
  Initialization/3(P0) -> Scope/1, P0/1
  Depth trigger/1(dT) -> dT/1
  Initialization/1(pulse) -> AND/2, Scope1/1
  AND/1 -> pulse/1

== system modello_completo_simulink2019b/Vehicle Model/Model Vehicle/Kinematic ==
  eta : Inport
  ni : Inport  Port=2
  Jac : MATLAB Function  TreatAsAtomicUnit=on
  Product : Product  Multiplication=Matrix(*)
  eta_dot : Outport  VectorParamsAs1DForOutWhenUnconnected=off
  wires:
  ni/1 -> Product/2
  Jac/1(J) -> Product/1
  eta/1 -> Jac/1(eta)
  Product/1 -> eta_dot/1

== system modello_completo_simulink2019b/Vehicle Model/Thrusters/T ==
  des rot : Inport
  ni : Inport  Port=2
  Demux : Demux  Outputs=7
  Demux1 : Demux  Outputs=7
  MATLAB Function : MATLAB Function  TreatAsAtomicUnit=on
  Mux : Mux  Inputs=7
  Thruster 1 : Subsystem
  Thruster 2 : Subsystem
  Thruster 3 : Subsystem
  Thruster 4 : Subsystem
  Thruster 5 : Subsystem
  Thruster 6 : Subsystem
  Thruster 7 : Subsystem
  T : Outport  VectorParamsAs1DForOutWhenUnconnected=off
  wires:
  Demux/1 -> Thruster 1/1(n [rad/s])
  Demux/2 -> Thruster 2/1(n [rad/s])
  Demux/3 -> Thruster 3/1(n [rad/s])
  Demux/4 -> Thruster 4/1(n [rad/s])
  Demux/5 -> Thruster 5/1(n [rad/s])
  Demux/6 -> Thruster 6/1(n [rad/s])
  Demux/7 -> Thruster 7/1(n [rad/s])
  des rot/1 -> Demux/1
  Thruster 7/1(T i) -> Mux/7
  Thruster 6/1(T i) -> Mux/6
  Thruster 5/1(T i) -> Mux/5
  Thruster 4/1(T i) -> Mux/4
  Thruster 3/1(T i) -> Mux/3
  Thruster 2/1(T i) -> Mux/2
  Thruster 1/1(T i) -> Mux/1
  Mux/1 -> T/1
  MATLAB Function/1(v_th) -> Demux1/1
  Demux1/1 -> Thruster 1/2(V [m/s])
  Demux1/2 -> Thruster 2/2(V [m/s])
  Demux1/3 -> Thruster 3/2(V [m/s])
  Demux1/4 -> Thruster 4/2(V [m/s])
  Demux1/5 -> Thruster 5/2(V [m/s])
  Demux1/6 -> Thruster 6/2(V [m/s])
  Demux1/7 -> Thruster 7/2(V [m/s])
  ni/1 -> MATLAB Function/1(ni)

== system modello_completo_simulink2019b/Navigation1/z_EKF/Trigger & Init/Depth trigger ==
  Meas_depth : Inport
  Demux : Demux  Outputs=2
  MATLAB Function : MATLAB Function  TreatAsAtomicUnit=on
  Sum : Sum  Inputs=|+-
  Terminator : Terminator
  count : Memory  InitialCondition=1
  prev_depth : Memory
  dT : Outport
  Pulse : Outport  Port=2
  wires:
  Sum/1 -> MATLAB Function/3(sum)
  prev_depth/1 -> Sum/2
  MATLAB Function/3(pulse) -> Pulse/1
  Demux/2 -> Terminator/1
  MATLAB Function/4(prev) -> prev_depth/1
  MATLAB Function/2(dT) -> dT/1
  Meas_depth/1 -> Demux/1
  count/1 -> MATLAB Function/1("count ")
  Demux/1 -> MATLAB Function/2(depth), Sum/1
  MATLAB Function/1(count) -> count/1

== system modello_completo_simulink2019b/Navigation1/z_EKF/Trigger & Init/Initialization ==
  Meas_depth : Inport
  Meas_pos : Inport  Port=2
  Demux1 : Demux  Outputs=[2 1]
  Demux2 : Demux  Outputs=2
  MATLAB Function1 : MATLAB Function  TreatAsAtomicUnit=on
  Scope3 : Scope
  Sum1 : Sum  Inputs=|+-
  Terminator2 : Terminator
  init_counter : Memory
  prev_pos : Memory  InitialCondition=zeros(2,1)
  store_depth : Memory  InitialCondition=zeros(num_cycle,1)
  store_gps : Memory  InitialCondition=zeros(2,num_cycle)
  pulse : Outport
  init : Outport  Port=2
  P0 : Outport  Port=3
  wires:
  Demux1/1 -> MATLAB Function1/3(gps), Sum1/1
  MATLAB Function1/4(P0) -> P0/1
  MATLAB Function1/3(init) -> init/1
  MATLAB Function1/2(pulse) -> pulse/1, Scope3/1
  init_counter/1 -> MATLAB Function1/1("init_counter ")
  Sum1/1 -> MATLAB Function1/5(diff_)
  Demux2/1 -> MATLAB Function1/2(depth)
  MATLAB Function1/6(gps_store) -> store_gps/1
  MATLAB Function1/1(init_counter) -> init_counter/1
  Demux2/2 -> Terminator2/1
  MATLAB Function1/7(depth_store) -> store_depth/1
  store_gps/1 -> MATLAB Function1/6(store_gps)
  store_depth/1 -> MATLAB Function1/7(store_depth)
  Meas_depth/1 -> Demux2/1
  MATLAB Function1/5(prev) -> prev_pos/1
  prev_pos/1 -> Sum1/2
  Meas_pos/1 -> Demux1/1
  Demux1/2 -> MATLAB Function1/4(GPS_flag)

== system modello_completo_simulink2019b/Vehicle Model/Thrusters/T/Thruster 1 ==
  note: n is the rotational speed of the thruster
      | V is the speed component of the water along the thruster axis
      |
      | n is saturated according to data
      | a dead zone is considered according to data
      | the thruster is characterised by 1st order dynamics (tau = 0.2s)
  n [rad/s] : Inport
  V [m/s] : Inport  Port=2
  Dead Zone : DeadZone  LowerValue=-dead_zone_limit  UpperValue=dead_zone_limit  SaturateOnIntegerOverflow=on
  MATLAB Function : MATLAB Function  TreatAsAtomicUnit=on
  Saturation : Saturate  UpperLimit=n_max  LowerLimit=-n_max
  Transfer Fcn : TransferFcn  Denominator=[0.2 1]
  T i : Outport
  wires:
  V [m/s]/1 -> MATLAB Function/2(V)
  Saturation/1 -> MATLAB Function/1(n)
  Transfer Fcn/1 -> Saturation/1
  Dead Zone/1 -> Transfer Fcn/1
  n [rad/s]/1 -> Dead Zone/1
  MATLAB Function/1(T) -> T i/1

== system modello_completo_simulink2019b/Vehicle Model/Thrusters/T/Thruster 2 ==
  note: n is the rotational speed of the thruster
      | V is the speed component of the water along the thruster axis
      |
      | n is saturated according to data
      | a dead zone is considered according to data
      | the thruster is characterised by 1st order dynamics (tau = 0.2s)
  n [rad/s] : Inport
  V [m/s] : Inport  Port=2
  Dead Zone : DeadZone  LowerValue=-dead_zone_limit  UpperValue=dead_zone_limit  SaturateOnIntegerOverflow=on
  MATLAB Function : MATLAB Function  TreatAsAtomicUnit=on
  Saturation : Saturate  UpperLimit=n_max  LowerLimit=-n_max
  Transfer Fcn : TransferFcn  Denominator=[0.2 1]
  T i : Outport
  wires:
  V [m/s]/1 -> MATLAB Function/2(V)
  Saturation/1 -> MATLAB Function/1(n)
  Transfer Fcn/1 -> Saturation/1
  Dead Zone/1 -> Transfer Fcn/1
  n [rad/s]/1 -> Dead Zone/1
  MATLAB Function/1(T) -> T i/1

== system modello_completo_simulink2019b/Vehicle Model/Thrusters/T/Thruster 3 ==
  note: n is the rotational speed of the thruster
      | V is the speed component of the water along the thruster axis
      |
      | n is saturated according to data
      | a dead zone is considered according to data
      | the thruster is characterised by 1st order dynamics (tau = 0.2s)
  n [rad/s] : Inport
  V [m/s] : Inport  Port=2
  Dead Zone : DeadZone  LowerValue=-dead_zone_limit  UpperValue=dead_zone_limit  SaturateOnIntegerOverflow=on
  MATLAB Function : MATLAB Function  TreatAsAtomicUnit=on
  Saturation : Saturate  UpperLimit=n_max  LowerLimit=-n_max
  Transfer Fcn : TransferFcn  Denominator=[0.2 1]
  T i : Outport
  wires:
  V [m/s]/1 -> MATLAB Function/2(V)
  Saturation/1 -> MATLAB Function/1(n)
  Transfer Fcn/1 -> Saturation/1
  Dead Zone/1 -> Transfer Fcn/1
  n [rad/s]/1 -> Dead Zone/1
  MATLAB Function/1(T) -> T i/1

== system modello_completo_simulink2019b/Vehicle Model/Thrusters/T/Thruster 4 ==
  note: n is the rotational speed of the thruster
      | V is the speed component of the water along the thruster axis
      |
      | n is saturated according to data
      | a dead zone is considered according to data
      | the thruster is characterised by 1st order dynamics (tau = 0.2s)
  n [rad/s] : Inport
  V [m/s] : Inport  Port=2
  Dead Zone : DeadZone  LowerValue=-dead_zone_limit  UpperValue=dead_zone_limit  SaturateOnIntegerOverflow=on
  MATLAB Function : MATLAB Function  TreatAsAtomicUnit=on
  Saturation : Saturate  UpperLimit=n_max  LowerLimit=-n_max
  Transfer Fcn : TransferFcn  Denominator=[0.2 1]
  T i : Outport
  wires:
  V [m/s]/1 -> MATLAB Function/2(V)
  Saturation/1 -> MATLAB Function/1(n)
  Transfer Fcn/1 -> Saturation/1
  Dead Zone/1 -> Transfer Fcn/1
  n [rad/s]/1 -> Dead Zone/1
  MATLAB Function/1(T) -> T i/1

== system modello_completo_simulink2019b/Vehicle Model/Thrusters/T/Thruster 5 ==
  note: n is the rotational speed of the thruster
      | V is the speed component of the water along the thruster axis
      |
      | n is saturated according to data
      | a dead zone is considered according to data
      | the thruster is characterised by 1st order dynamics (tau = 0.2s)
  n [rad/s] : Inport
  V [m/s] : Inport  Port=2
  Dead Zone : DeadZone  LowerValue=-dead_zone_limit  UpperValue=dead_zone_limit  SaturateOnIntegerOverflow=on
  MATLAB Function : MATLAB Function  TreatAsAtomicUnit=on
  Saturation : Saturate  UpperLimit=n_max  LowerLimit=-n_max
  Transfer Fcn : TransferFcn  Denominator=[0.2 1]
  T i : Outport
  wires:
  V [m/s]/1 -> MATLAB Function/2(V)
  Saturation/1 -> MATLAB Function/1(n)
  Transfer Fcn/1 -> Saturation/1
  Dead Zone/1 -> Transfer Fcn/1
  n [rad/s]/1 -> Dead Zone/1
  MATLAB Function/1(T) -> T i/1

== system modello_completo_simulink2019b/Vehicle Model/Thrusters/T/Thruster 6 ==
  note: n is the rotational speed of the thruster
      | V is the speed component of the water along the thruster axis
      |
      | n is saturated according to data
      | a dead zone is considered according to data
      | the thruster is characterised by 1st order dynamics (tau = 0.2s)
  n [rad/s] : Inport
  V [m/s] : Inport  Port=2
  Dead Zone : DeadZone  LowerValue=-dead_zone_limit  UpperValue=dead_zone_limit  SaturateOnIntegerOverflow=on
  MATLAB Function : MATLAB Function  TreatAsAtomicUnit=on
  Saturation : Saturate  UpperLimit=n_max  LowerLimit=-n_max
  Transfer Fcn : TransferFcn  Denominator=[0.2 1]
  T i : Outport
  wires:
  V [m/s]/1 -> MATLAB Function/2(V)
  Saturation/1 -> MATLAB Function/1(n)
  Transfer Fcn/1 -> Saturation/1
  Dead Zone/1 -> Transfer Fcn/1
  n [rad/s]/1 -> Dead Zone/1
  MATLAB Function/1(T) -> T i/1

== system modello_completo_simulink2019b/Vehicle Model/Thrusters/T/Thruster 7 ==
  note: n is the rotational speed of the thruster
      | V is the speed component of the water along the thruster axis
      |
      | n is saturated according to data
      | a dead zone is considered according to data
      | the thruster is characterised by 1st order dynamics (tau = 0.2s)
  n [rad/s] : Inport
  V [m/s] : Inport  Port=2
  Dead Zone : DeadZone  LowerValue=-dead_zone_limit  UpperValue=dead_zone_limit  SaturateOnIntegerOverflow=on
  MATLAB Function : MATLAB Function  TreatAsAtomicUnit=on
  Saturation : Saturate  UpperLimit=n_max  LowerLimit=-n_max
  Transfer Fcn : TransferFcn  Denominator=[0.2 1]
  T i : Outport
  wires:
  V [m/s]/1 -> MATLAB Function/2(V)
  Saturation/1 -> MATLAB Function/1(n)
  Transfer Fcn/1 -> Saturation/1
  Dead Zone/1 -> Transfer Fcn/1
  n [rad/s]/1 -> Dead Zone/1
  MATLAB Function/1(T) -> T i/1

== matlab function modello_completo_simulink2019b/Vehicle Model/Model Vehicle/D ==
  data: ni_r input; F_d output; rho input
function F_d = D_forces(ni_r, rho)
    ni_lin = ni_r(1:3);
    ni_ang = ni_r(4:6);
    a = 0.35;
    b = a;
    c = 0.19;
    A_ab = pi*a*b;      % moto lin lungo z; rotatorio intorno a x e y
    A_bc = pi*b*c;      % moto lin lungo x; rotatorio intorno a z
    A_ac = pi*a*c;      % moto lin lungo y
%     C_d  =  0.0489;
%     D_coeff = -1/2*rho*C_d*diag([A_bc, A_ac, A_ab, A_bc, A_ac, A_ab]);
%     F_d = D_coeff*(abs(ni_r).*ni_r);
    visc = 0.001;       % Pa*s (per una temperatura di 20° e rho = 1030)
    vmax = 0.3;
    Di = 0.7;
    Re = Di/(visc/rho)*vmax; % Re = 2*1e5
    Cd = 0.49;
    rm_z = 4*c/(3*pi);
    rm_xy = 4*a/(3*pi);
    D_lin = -1/2*rho*Cd*diag([A_bc, A_ac, A_ab])*(abs(ni_lin).*ni_lin);
    D_ang = -1/2*rho*Cd*diag([rm_xy^3*A_ab, rm_xy^3*A_ab, rm_z^3*A_bc])*(abs(ni_ang).*ni_ang);
    F_d = [D_lin; D_ang];
end

== matlab function modello_completo_simulink2019b/Vehicle Model/Model Vehicle/C ==
  data: ni_r input; F_c output; M input
function F_c = C(ni_r, M)
    ni = ni_r;
    M11 = M(1:3,1:3);
    M22 = M(4:6,4:6);
    ni1 = ni(1:3);
    ni2 = ni(4:6);
    C11 = zeros(3,3);
    s1 = M11*ni1;
    C12 = - [0 -s1(3) s1(2); s1(3) 0 -s1(1); -s1(2) s1(1) 0];
    C21 = C12;
    s2 = M22*ni2;
    C22 = - [0 -s2(3) s2(2); s2(3) 0 -s2(1); -s2(2) s2(1) 0];
    F_c = [C11 C12; C21 C22]*ni_r;
end

== matlab function modello_completo_simulink2019b/Vehicle Model/Model Vehicle/grav ==
  data: rho input; eta input; F_g output
function F_g = grav(rho, eta)
    eta2 = eta(4:6);
    g = 9.81;   
    a = 0.35;
    b = a;
    c = 0.19;
    massa = 100;
    if eta(3) >= c
       V = 4/3*pi*a*b*c;
    else
       V = 4/3*pi*a*b*c - (pi*a*b/(3*c^2))*((eta(3)-c)^2)*(3*c - abs(eta(3) - c)); 
    end
    W = massa*g;
    B = rho*V*g;
    J = Jac(eta2);
    J1 = J(1:3,1:3);
    J2 = J(4:6,4:6);
    f_g = inv(J1)*[0; 0; W];
    f_b = inv(J1)*[0; 0; -B];
    r_g = [0; 0; 0];
    r_b = [0; 0; -c/2];
    %TODO: inserire un contributo nullo di forza quando siamo a galla (?)
%     if eta(3) < 0
%        F_g = [0; 0; 0; 0; 0; 0];
%     else
    F_g = -[f_g + f_b; cross(r_g,f_g) + cross(r_b,f_b)];
%     end
end

== matlab function modello_completo_simulink2019b/Vehicle Model/Model Vehicle/Kinematic/Jac ==
  data: eta input; J output
function J = Jac(eta)
    eta2 = eta(4:6);
    phi = eta2(1);
    theta = eta2(2);
    psi = eta2(3);
    Rx = [1 0 0; 0 cos(phi) sin(phi); 0 -sin(phi) cos(phi)];
    Ry = [cos(theta) 0 -sin(theta); 0 1 0; sin(theta) 0 cos(theta)];
    Rz = [cos(psi) sin(psi) 0; -sin(psi) cos(psi) 0; 0 0 1];
    J1 = Rz'*Ry'*Rx';
    J2 = [1 sin(phi)*tan(theta) cos(phi)*tan(theta); ...
        0 cos(phi) -sin(phi); ...
        0 sin(phi)/cos(theta) cos(phi)/cos(theta)];
    J = blkdiag(J1, J2);
end

== matlab function modello_completo_simulink2019b/Vehicle Model/Thrusters/T/Thruster 1/MATLAB Function ==
  data: n input; T output; V input; D parameter; omega parameter; a1 parameter; a2 parameter; alpha1 parameter; alpha2 parameter
function T = thrusterModel(n, V, D, omega, a1, a2, alpha1, alpha2)

Va = (1-omega) * V;     % Advancement velocity at the propeller
J0 = Va/(n*D);          % Advancement Coefficient

if J0 > -alpha1/alpha2  % Out of linearity domain (right side)
    T = 0;              % A null generated thrust is assumed
    
elseif J0 < 0           % Out of linearity domain (left side)
    T = a1*abs(n)*n;    % Bollard thrust is assumed

else                    % Within the linearity domain
    T = a1*abs(n)*n - a2*abs(n)*V;
end

== matlab function modello_completo_simulink2019b/Vehicle Model/Thrusters/T/Thruster 2/MATLAB Function ==
  data: n input; T output; V input; D parameter; omega parameter; a1 parameter; a2 parameter; alpha1 parameter; alpha2 parameter
function T = thrusterModel(n, V, D, omega, a1, a2, alpha1, alpha2)

Va = (1-omega) * V;     % Advancement velocity at the propeller
J0 = Va/(n*D);          % Advancement Coefficient

if J0 > -alpha1/alpha2  % Out of linearity domain (right side)
    T = 0;              % A null generated thrust is assumed
    
elseif J0 < 0           % Out of linearity domain (left side)
    T = a1*abs(n)*n;    % Bollard thrust is assumed

else                    % Within the linearity domain
    T = a1*abs(n)*n - a2*abs(n)*V;
end

== matlab function modello_completo_simulink2019b/Vehicle Model/Thrusters/T/Thruster 3/MATLAB Function ==
  data: n input; T output; V input; D parameter; omega parameter; a1 parameter; a2 parameter; alpha1 parameter; alpha2 parameter
function T = thrusterModel(n, V, D, omega, a1, a2, alpha1, alpha2)

Va = (1-omega) * V;     % Advancement velocity at the propeller
J0 = Va/(n*D);          % Advancement Coefficient

if J0 > -alpha1/alpha2  % Out of linearity domain (right side)
    T = 0;              % A null generated thrust is assumed
    
elseif J0 < 0           % Out of linearity domain (left side)
    T = a1*abs(n)*n;    % Bollard thrust is assumed

else                    % Within the linearity domain
    T = a1*abs(n)*n - a2*abs(n)*V;
end

== matlab function modello_completo_simulink2019b/Vehicle Model/Thrusters/T/Thruster 4/MATLAB Function ==
  data: n input; T output; V input; D parameter; omega parameter; a1 parameter; a2 parameter; alpha1 parameter; alpha2 parameter
function T = thrusterModel(n, V, D, omega, a1, a2, alpha1, alpha2)

Va = (1-omega) * V;     % Advancement velocity at the propeller
J0 = Va/(n*D);          % Advancement Coefficient

if J0 > -alpha1/alpha2  % Out of linearity domain (right side)
    T = 0;              % A null generated thrust is assumed
    
elseif J0 < 0           % Out of linearity domain (left side)
    T = a1*abs(n)*n;    % Bollard thrust is assumed

else                    % Within the linearity domain
    T = a1*abs(n)*n - a2*abs(n)*V;
end

== matlab function modello_completo_simulink2019b/Vehicle Model/Thrusters/T/Thruster 5/MATLAB Function ==
  data: n input; T output; V input; D parameter; omega parameter; a1 parameter; a2 parameter; alpha1 parameter; alpha2 parameter
function T = thrusterModel(n, V, D, omega, a1, a2, alpha1, alpha2)

Va = (1-omega) * V;     % Advancement velocity at the propeller
J0 = Va/(n*D);          % Advancement Coefficient

if J0 > -alpha1/alpha2  % Out of linearity domain (right side)
    T = 0;              % A null generated thrust is assumed
    
elseif J0 < 0           % Out of linearity domain (left side)
    T = a1*abs(n)*n;    % Bollard thrust is assumed

else                    % Within the linearity domain
    T = a1*abs(n)*n - a2*abs(n)*V;
end

== matlab function modello_completo_simulink2019b/Vehicle Model/Thrusters/T/Thruster 6/MATLAB Function ==
  data: n input; T output; V input; D parameter; omega parameter; a1 parameter; a2 parameter; alpha1 parameter; alpha2 parameter
function T = thrusterModel(n, V, D, omega, a1, a2, alpha1, alpha2)

Va = (1-omega) * V;     % Advancement velocity at the propeller
J0 = Va/(n*D);          % Advancement Coefficient

if J0 > -alpha1/alpha2  % Out of linearity domain (right side)
    T = 0;              % A null generated thrust is assumed
    
elseif J0 < 0           % Out of linearity domain (left side)
    T = a1*abs(n)*n;    % Bollard thrust is assumed

else                    % Within the linearity domain
    T = a1*abs(n)*n - a2*abs(n)*V;
end
